simulink library "tm4c1294npdt"  (R2013b)
settings: Solver=ode45  StartTime=0.0  StopTime=10.0  RelTol=1e-3
libraries: tm4c1294npdt x2
settings Model: Creator=Q365198  LastModifiedBy=Q365198

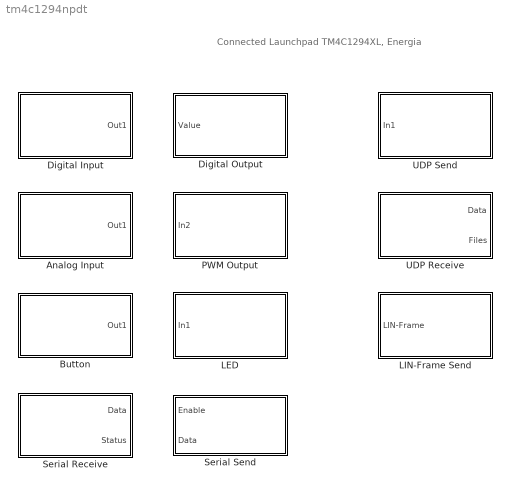
== system tm4c1294npdt ==
  note: Connected Launchpad TM4C1294XL, Energia
  Analog Input : Subsystem  mask(Energia Analog Input){popup_pin=14, pin=2, SampleTime=-1}
      mask prompts: popup_pin "Analog Input Pin:"; pin "Analog Pin"; SampleTime "Sample Time (-1 for inherited):"
      mask help:
      | Measure the voltage of a specified analog input pin. The block represents the voltage as a digital value (0-1023, minimum to maximum).
      |
      | Enter the number of the analog input pin. Do not assign the same pin number to multiple blocks within a model.
      mask TypeOptions popup_pin: 2 | 6 | 7 | 14 | 15 | 23 | 24 | 25 | 26 | 27 | 42 | 45 | 46 | 63 | 64 | 65 | 66 | 67 | 68 | 87
      mask Callback popup_pin:
      | thisBlock = gcb();
      | 
      | thisVarState = get_param(thisBlock, 'popup_pin');
      | set_param(thisBlock, 'pin', thisVarState);
      mask Display:
      | pic=imread('analogio.png');image(pic,[0.32 0.25 0.35 0.55]);
      | str = sprintf('Pin %i', pin);
      | text(0.5, 0.15, str, 'horizontalAlignment', 'center');
      | color('blue');
      | text(0.35, 0.87, 'TM4C1294XL', 'horizontalAlignment', 'left');
      | color('black');
  Button : Subsystem  mask(TM4C1294XL User Buttons){popup_pin=USR_SW1, pin=85, mode_popup=INPUT_PULLUP, mode=3, SampleTime=-1}
      mask prompts: popup_pin "User Button:"; pin "PinMode"; mode_popup "Input Mode:"; SampleTime "Sample Time (-1 for inherited):"
      mask help:
      | Read the logical value of a specified user Button on the TM4C1294XL Connected Launchpad.
      |
      | Choose available Buttons using the dropdown menu. Do not assign identical Buttons to more than one block (Fuctionality not guaranteed).
      mask TypeOptions popup_pin: USR_SW1 | USR_SW2
      mask Callback popup_pin:
      | thisBlock = gcb();
      | 
      | thisVarState = get_param(thisBlock, 'popup_pin');
      | if strcmp(thisVarState, 'USR_SW1')
      |     set_param(thisBlock, 'pin', '85');
      | elseif strcmp(thisVarState, 'USR_SW2')
      |     set_param(thisBlock, 'pin', '86');
      | end
      mask TypeOptions mode_popup: INPUT | INPUT_PULLDOWN | INPUT_PULLUP
      mask Callback mode_popup:
      | thisBlock = gcb();
      | 
      | thisVarState = get_param(thisBlock, 'mode_popup');
      | if strcmp(thisVarState, 'INPUT')
      |     set_param(thisBlock, 'mode', '1');
      | elseif strcmp(thisVarState, 'INPUT_PULLDOWN')
      |     set_param(thisBlock, 'mode', '2');
      | elseif strcmp(thisVarState, 'INPUT_PULLUP')
      |     set_param(thisBlock, 'mode', '3');
      | end
      mask Display:
      | pic=imread('push_button.jpg');image(pic,[0.32 0.20 0.35 0.55]);
      | str = sprintf('Pin %i', pin);
      | text(0.5, 0.15, str, 'horizontalAlignment', 'center');
      | color('blue');
      | text(0.35, 0.87, 'TM4C1294XL', 'horizontalAlignment', 'left');
      | color('black');
      | 
      | % Output Label
      | MaskValues=get_param(gcbh, 'MaskValues');
      | switch MaskValues{3}
      |     case 'INPUT'
      |         label = 'IN';
      |     case 'INPUT_PULLDOWN'
      |         label = 'IN_PD';
      |     case 'INPUT_PULLUP'
      |         label = 'IN_PU';
      |     otherwise
      |         label = '';
      | end
      | port_label('output',1,label);
  Digital Input : Subsystem  mask(Energia Digital Input){pin=2, mode_popup=INPUT, mode=1, SampleTime=-1}
      mask prompts: pin "Input Pin Number:"; mode_popup "Input Mode:"; SampleTime "Sample Time (-1 for inherited):"
      mask help:
      | Get the logical value of a specified digital input pin.
      |
      | Enter the number of the digital input pin. Do not assign the same pin number to multiple blocks within a model.
      mask TypeOptions mode_popup: INPUT | INPUT_PULLDOWN | INPUT_PULLUP
      mask Callback mode_popup:
      | thisBlock = gcb();
      | 
      | thisVarState = get_param(thisBlock, 'mode_popup');
      | if strcmp(thisVarState, 'INPUT')
      |     set_param(thisBlock, 'mode', '1');
      | elseif strcmp(thisVarState, 'INPUT_PULLDOWN')
      |     set_param(thisBlock, 'mode', '2');
      | elseif strcmp(thisVarState, 'INPUT_PULLUP')
      |     set_param(thisBlock, 'mode', '3');
      | end
      mask Display:
      | pic=imread('digitalio.png');image(pic,[0.32 0.25 0.35 0.55]);
      | str = sprintf('Pin %i', pin);
      | text(0.5, 0.15, str, 'horizontalAlignment', 'center');
      | color('blue');
      | text(0.35, 0.87, 'TM4C1294XL', 'horizontalAlignment', 'left');
      | color('black');
      | 
      | % Output Label
      | MaskValues=get_param(gcbh, 'MaskValues');
      | switch MaskValues{2}
      |     case 'INPUT'
      |         label = 'IN';
      |     case 'INPUT_PULLDOWN'
      |         label = 'IN_PD';
      |     case 'INPUT_PULLUP'
      |         label = 'IN_PU';
      | end
      | port_label('output',1,label);
  Digital Output : Subsystem  mask(Energia Digital Output){pin=82, SampleTime=-1}
      mask prompts: pin "Output Pin Number"; SampleTime "Sample Time (-1 for inherited):"
      mask help:
      | Set the logical value of a specified digital output pin.
      |
      | Enter the number of the digital output pin. Do not assign the same pin number to multiple blocks within a model.
      mask Display:
      | pic=imread('digitalio.png');image(pic,[0.32 0.25 0.35 0.55]);
      | str = sprintf('Pin %i', pin);
      | text(0.5, 0.15, str, 'horizontalAlignment', 'center');
      | color('blue');
      | text(0.35, 0.87, 'TM4C1294XL', 'horizontalAlignment', 'left');
      | color('black');
  LED : Subsystem  mask(TM4C1294XL User LEDs){popup_led=LED1, pin=81, SampleTime=-1}
      mask prompts: popup_led "User LEDs:"; SampleTime "Sample Time (-1 for inherited):"
      mask help:
      | Set the logical value of a specified user LED on the TM4C1294XL Connected Launchpad.
      |
      | Choose available LEDs using the dropdown menu. Do not assign identical LEDs to more than one block (Fuctionality not guaranteed).
      mask TypeOptions popup_led: LED1 | LED2 | LED3 | LED4
      mask Callback popup_led:
      | thisBlock = gcb();
      | 
      | thisVarState = get_param(thisBlock, 'popup_led');
      | if strcmp(thisVarState, 'LED1')
      |     set_param(thisBlock, 'pin', '81');
      | elseif strcmp(thisVarState, 'LED2')
      |     set_param(thisBlock, 'pin', '82');
      | elseif strcmp(thisVarState, 'LED3')
      |     set_param(thisBlock, 'pin', '83');
      | elseif strcmp(thisVarState, 'LED4')
      |     set_param(thisBlock, 'pin', '84');
      | end
      mask Display:
      | pic=imread('led_green.png');image(pic,[0.32 0.20 0.35 0.55]);
      | str = sprintf('Pin %i', pin);
      | text(0.5, 0.15, str, 'horizontalAlignment', 'center');
      | color('blue');
      | text(0.35, 0.87, 'TM4C1294XL', 'horizontalAlignment', 'left');
      | color('black');
  LIN-Frame Send : Subsystem  mask(LIN-Frame Send){portPopup=2, port=2, baudPopup=19200, baud=19200, txPin=57, SampleTime=-1}
      mask prompts: portPopup "Serial Port:"; baudPopup "Baudrate:"; SampleTime "Sample Time (-1 for inherited):"
      mask help:
      | This block is acutally sending complete LIN-Frames using baud speed and your defined UART port.
      |
      | REMEMBER: You have to input a byte stream which is representing a LIN-Frame but WITHOUT the "Break field".
      | -> The Bytestream should contain:
      | 1. Sync Field (0x55), 1 Byte
      | 2. Identifier (EventID, care about Parity), 1 Byte
      | 3. Databytes, 1 - 8 Bytes
      | 4. Checksum, 1 Byte
      mask TypeOptions portPopup: 2 | 3 | 4 | 5 | 6 | 7
      mask Callback portPopup:
      | thisBlock = gcb();
      | 
      | thisVarState = get_param(thisBlock, 'portPopup');
      | set_param(thisBlock, 'port', thisVarState);
      | 
      | switch thisVarState
      |     case '2'
      |         set_param(thisBlock, 'txPin', '57');
      |     case '3'
      |         set_param(thisBlock, 'txPin', '70');
      |     case '4'
      |         set_param(thisBlock, 'txPin', '66');
      |     case '5'
      |         set_param(thisBlock, 'txPin', '8');
      |     case '6'
      |         set_param(thisBlock, 'txPin', '44');
      |     case '7'
      |         set_param(thisBlock, 'txPin', '4');
      |     otherwise
      |         set_param(thisBlock, 'txPin', '57');
      | end
      mask TypeOptions baudPopup: 300 | 1200 | 2400 | 4800 | 9600 | 14400 | 19200 | 28800 | 38400 | 57600 | 76800 | 115200
      mask Callback baudPopup:
      | thisBlock = gcb();
      | 
      | thisVarState = get_param(thisBlock, 'baudPopup');
      | set_param(thisBlock, 'baud', thisVarState);
      mask Display:
      | pic=imread('Lin_Logo.jpg');image(pic,[0.50 0.10 0.45 0.65]);
      | 
      | color('blue');
      | text(0.38, 0.87, 'TM4C1294XL', 'horizontalAlignment', 'left');
      | 
      | color('red')
      | str = sprintf('UART%i',port);
      | text(0.02, 0.87, str,'horizontalAlignment', 'left');
      | color('black');
      | 
      | port_label('input', 1, 'LIN-Frame');
  PWM Output : Subsystem  mask(Energia PWM Output){popup_pin=7, pin=7, SampleTime=-1}
      mask prompts: popup_pin "PWM Output Pin:"; pin "PWM Output Pin:"; SampleTime "Sample Time (-1 for inherited):"
      mask help:
      | Generate square waveform on the specified analog output pin. The block input controls the duty cycle of the square waveform. An input value of 0 produces a 0 percent duty cycle, and an input value of 255 produces a 100 percent duty cycle. The frequency of the waveform is constant at approximately 490 Hz.
      |
      | Enter the number of the analog output pin (7, 9, 10, 14, 15, 19, 27-30, 35, 36, 42, 45, 46, 51, 57, 59, 69, 70, 75 - 77, 87, 90, 91). Do not assign the same pin number to multiple blocks within a model.
      mask TypeOptions popup_pin: 7 | 9 | 10 | 14 | 15 | 19 | 27 | 28 | 29 | 30 | 35 | 36 | 42 | 45 | 46 | 51 | 57 | 59 | 69 | 70 | 75 | 76 | 77 | 87 | 90 | 91
      mask Callback popup_pin:
      | thisBlock = gcb();
      | 
      | thisVarState = get_param(thisBlock, 'popup_pin');
      | set_param(thisBlock, 'pin', thisVarState);
      mask Display:
      | pic=imread('analogoutpwm.png');image(pic,[0.32 0.25 0.35 0.55]);
      | str = sprintf('Pin %i', pin);
      | text(0.5, 0.15, str, 'horizontalAlignment', 'center');
      | color('blue');
      | text(0.35, 0.87, 'TM4C1294XL', 'horizontalAlignment', 'left');
      | color('black');
  Serial Receive : Subsystem  mask(Energia Serial Receive){portPopup=1, port=1, baudPopup=9600, baud=9600, bufferSize=32, SampleTime=-1}
      mask prompts: portPopup "UART-Port (0 = flash/debug):"; baudPopup "Baudrate:"; bufferSize "Receive Buffer Size (1...64):"; SampleTime "Sample Time (-1 for inherited):"
      mask help:
      | Get bytes of data from the specified serial port and write it to the Data block output. Maximum Datasize can be defined (64 Bytes = Hardware Buffer).
      |
      | If data is received, Status block output gives the size of the received data. If data is not received, Status is equal 0.
      |
      | Do not assign the same port to more than one Serial Receive block. Please remeber that UART0 is normally used for debug/flash and external mode.
      mask TypeOptions portPopup: 0 | 1 | 2 | 3 | 4 | 5 | 6 | 7
      mask Callback portPopup:
      | thisBlock = gcb();
      | 
      | thisVarState = get_param(thisBlock, 'portPopup');
      | set_param(thisBlock, 'port', thisVarState);
      mask TypeOptions baudPopup: 300 | 1200 | 2400 | 4800 | 9600 | 14400 | 19200 | 28800 | 38400 | 57600 | 76800 | 115200
      mask Callback baudPopup:
      | thisBlock = gcb();
      | 
      | thisVarState = get_param(thisBlock, 'baudPopup');
      | set_param(thisBlock, 'baud', thisVarState);
      mask Display:
      | pic=imread('serial.png');image(pic,[0.28 0.18 0.45 0.65]);
      | 
      | str = sprintf('UART%i', (portPopup-1));
      | text(0.5, 0.15, str, 'horizontalAlignment', 'center');
      | color('blue');
      | text(0.35, 0.87, 'TM4C1294XL', 'horizontalAlignment', 'left');
      | color('black');
      | 
      | color('blue');
      | text(0.35, 0.87, 'TM4C1294XL', 'horizontalAlignment', 'left');
      | color('black');
      | 
      | str = sprintf('Data[%i]', bufferSize);
      | port_label('output', 1, str);
      | port_label('output', 2, 'Status');
  Serial Send : Subsystem  mask(Energia Serial Write){portPopup=1, port=1, baudPopup=9600, baud=9600, SampleTime=-1}
      mask prompts: portPopup "UART-Port (0 = flash/debug):"; baudPopup "Baudrate:"; SampleTime "SampleTime (-1 for inherited):"
      mask help:
      | Write bytes of data to the specified serial portt. Maximum Datasize should be 64 Bytes (Hardware Buffer).
      |
      | Do not assign the same port to more than one Serial Receive block. Please remeber that UART0 is normally used for debug/flash and external mode.
      mask TypeOptions portPopup: 0 | 1 | 2 | 3 | 4 | 5 | 6 | 7
      mask Callback portPopup:
      | thisBlock = gcb();
      | 
      | thisVarState = get_param(thisBlock, 'portPopup');
      | set_param(thisBlock, 'port', thisVarState);
      mask TypeOptions baudPopup: 300 | 1200 | 2400 | 4800 | 9600 | 14400 | 19200 | 28800 | 38400 | 57600 | 76800 | 115200
      mask Callback baudPopup:
      | thisBlock = gcb();
      | 
      | thisVarState = get_param(thisBlock, 'baudPopup');
      | set_param(thisBlock, 'baud', thisVarState);
      mask Display:
      | pic=imread('serial.png');image(pic,[0.28 0.18 0.45 0.65]);
      | 
      | str = sprintf('UART%i', (portPopup-1));
      | text(0.5, 0.15, str, 'horizontalAlignment', 'center');
      | color('blue');
      | text(0.35, 0.87, 'TM4C1294XL', 'horizontalAlignment', 'left');
      | color('black');
      | 
      | color('blue');
      | text(0.35, 0.87, 'TM4C1294XL', 'horizontalAlignment', 'left');
      | color('black');
      | 
      | str = sprintf('Data');
      | port_label('input', 2, str);
      | port_label('input', 1, 'Enable');
  UDP Receive : Subsystem  mask(Energia UDP Send){localPort=8000, simVectorSize=8, SampleTime=-1}
      mask prompts: localPort "Local Port:"; simVectorSize "Output Vector Size (1-500)"; SampleTime "Sample time (-1 for inherited):"
      mask help: Configure TCP/IP stack to send UDP messages to a remote interface identified by IP address and IP port pair.
      mask Display:
      | pic=imread('ethernetshield.png');image(pic,[0.32 0.25 0.35 0.55]);text(0.5, 0.15, 'Pin 9', 'horizontalAlignment', 'center');
      | color('blue');
      | text(0.35, 0.87, 'TM4C1294XL', 'horizontalAlignment', 'left');
      | color('black');
  UDP Send : Subsystem  mask(Energia UDP Send){remoteIPOctetString=192.168.0.5, remotePort=8888, localport=8000, remoteIP1=192, remoteIP2=168, remoteIP3=0, remoteIP4=5, SampleTime=-1}
      mask prompts: remoteIPOctetString "Remote IP Address:"; remotePort "Remote Port:"; localport "Local Port:"; remoteIP1 "Remote IP First"; remoteIP2 "Remote IP Second"; remoteIP3 "Remote IP Third"; remoteIP4 "Remote IP Fourth"; SampleTime "Sample time (-1 for inherited):"
      mask help: Configure TCP/IP stack to send UDP messages to a remote interface identified by IP address and IP port pair.
      mask Callback remoteIPOctetString:
      | thisBlock = gcb();
      | 
      | thisVarState = get_param(thisBlock, 'remoteIPOctetString');
      | parts = strsplit(thisVarState, '.');
      | set_param(thisBlock, 'remoteIP1', parts{1});
      | set_param(thisBlock, 'remoteIP2', parts{2});
      | set_param(thisBlock, 'remoteIP3', parts{3});
      | set_param(thisBlock, 'remoteIP4', parts{4});
      mask Display:
      | pic=imread('ethernetshield.png');image(pic,[0.32 0.25 0.35 0.55]);text(0.5, 0.15, 'Pin 9', 'horizontalAlignment', 'center');
      | color('blue');
      | text(0.35, 0.87, 'TM4C1294XL', 'horizontalAlignment', 'left');
      | color('black');

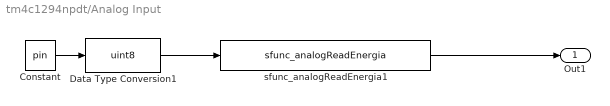
== system tm4c1294npdt/Analog Input ==
  Constant : Constant  Value=pin
  Data Type Conversion1 : DataTypeConversion  OutDataTypeStr=uint8  SaturateOnIntegerOverflow=on
  sfunc_analogReadEnergia1 : S-Function  FunctionName=sfunc_analogReadEnergia  Parameters=SampleTime  EnableBusSupport=off  mask(Legacy Function){SFunctionSpec=int16 y1 = analogReadEnergia(uint8 u1), SampleTime=SampleTime, ShowSpec=on}
      mask prompts: SampleTime "Sample time (-1 for inherited):"; ShowSpec "Display function specification"
      mask help:
      | This block allows you to call the legacy functions specified by the following Legacy Code Tool definition:
      | def.SFunctionName = 'sfunc_analogReadEnergia';
      | def.OutputFcnSpec = 'int16 y1 = analogReadEnergia(uint8 u1)';
      | def.HeaderFiles = {'gpioEnergia.h'};
      | def.SourceFiles = {'gpioEnergia.c'};
      | def.IncPaths = {'C:\MATLAB\SupportPackages\R2013b\TM4C1294NPDT\blocks\src\'};
      | def.SrcPaths = {'C:\MATLAB\SupportPackages\R2013b\TM4C1294NPDT\blocks\src\'};
      | def.SampleTime = 'parameterized';
      mask Help: <p>This block was generated automatically by the Legacy Code Tool. For detailed help on this tool, call<a href="matlab:legacy_code('help')"> legacy_code('help')</a>.</p>
      mask Callback ShowSpec:
      | if strcmp(get_param(gcbh, 'ShowSpec'), 'on')
      |   set_param(gcbh, 'MaskDisplay', sprintf('fprintf(''%s'');', get_param(gcbh, 'SFunctionSpec')));
      | else
      |   set_param(gcbh, 'MaskDisplay', sprintf('fprintf(''%s'');', get_param(gcbh, 'FunctionName')));
      | end
      mask Display: fprintf('int16 y1 = analogReadEnergia(uint8 u1)');
  Out1 : Outport
  wires:
  sfunc_analogReadEnergia1/1 -> Out1/1
  Constant/1 -> Data Type Conversion1/1
  Data Type Conversion1/1 -> sfunc_analogReadEnergia1/1

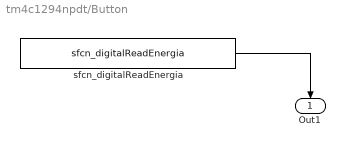
== system tm4c1294npdt/Button ==
  sfcn_digitalReadEnergia : tm4c1294npdt/Digital Input/sfcn_digitalReadEnergia  SFunctionSpec=uint8 y1 = digitalReadEnergia(uint8 p1)  SParameter1=pin  SParameter2=mode  SampleTime=SampleTime  ShowSpec=on
  Out1 : Outport
  wires:
  sfcn_digitalReadEnergia/1 -> Out1/1

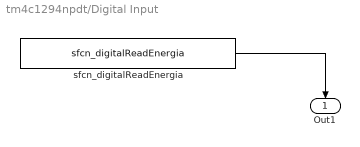
== system tm4c1294npdt/Digital Input ==
  sfcn_digitalReadEnergia : S-Function  FunctionName=sfcn_digitalReadEnergia  Parameters=SParameter1, SParameter2, SampleTime  EnableBusSupport=off  mask(Legacy Function){SFunctionSpec=uint8 y1 = digitalReadEnergia(uint8 p1), SParameter1=pin, SParameter2=mode, SampleTime=SampleTime, ShowSpec=on}
      mask prompts: SParameter1 "P1:"; SParameter2 "P2:"; SampleTime "Sample time (-1 for inherited):"; ShowSpec "Display function specification"
      mask help:
      | This block allows you to call the legacy functions specified by the following Legacy Code Tool definition:
      | def.SFunctionName = 'sfcn_digitalReadEnergia';
      | def.OutputFcnSpec = 'uint8 y1 = digitalReadEnergia(uint8 p1)';
      | def.StartFcnSpec = 'void digitalModeInitialize(uint8 p1, uint8 p2)';
      | def.HeaderFiles = {'gpioEnergia.h'};
      | def.SourceFiles = {'gpioEnergia.c'};
      | def.IncPaths = {'C:\MATLAB\SupportPackages\R2013b\TM4C1294NPDT\blocks\src\'};
      | def.SrcPaths = {'C:\MATLAB\SupportPackages\R2013b\TM4C1294NPDT\blocks\src\'};
      | def.SampleTime = 'parameterized';
      mask Help: <p>This block was generated automatically by the Legacy Code Tool. For detailed help on this tool, call<a href="matlab:legacy_code('help')"> legacy_code('help')</a>.</p>
      mask Callback ShowSpec:
      | if strcmp(get_param(gcbh, 'ShowSpec'), 'on')
      |   set_param(gcbh, 'MaskDisplay', sprintf('fprintf(''%s'');', get_param(gcbh, 'SFunctionSpec')));
      | else
      |   set_param(gcbh, 'MaskDisplay', sprintf('fprintf(''%s'');', get_param(gcbh, 'FunctionName')));
      | end
      mask Display: fprintf('uint8 y1 = digitalReadEnergia(uint8 p1)');
  Out1 : Outport
  wires:
  sfcn_digitalReadEnergia/1 -> Out1/1

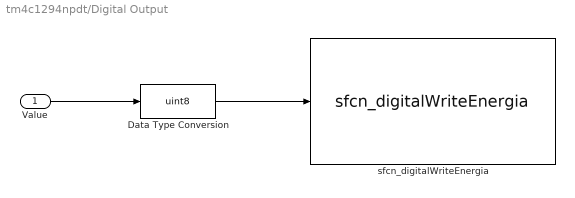
== system tm4c1294npdt/Digital Output ==
  Value : Inport
  Data Type Conversion : DataTypeConversion  OutDataTypeStr=uint8  SaturateOnIntegerOverflow=on
  sfcn_digitalWriteEnergia : S-Function  FunctionName=sfcn_digitalWriteEnergia  Parameters=SParameter1, SParameter2, SampleTime  EnableBusSupport=off  mask(Legacy Function){SFunctionSpec=void digitalWriteEnergia(uint8 p1, uint8 u1), SParameter1=pin, SParameter2=4, SampleTime=SampleTime, ShowSpec=on}
      mask prompts: SParameter1 "P1:"; SParameter2 "P2:"; SampleTime "Sample time (-1 for inherited):"; ShowSpec "Display function specification"
      mask help:
      | This block allows you to call the legacy functions specified by the following Legacy Code Tool definition:
      | def.SFunctionName = 'sfcn_digitalWriteEnergia';
      | def.OutputFcnSpec = 'void digitalWriteEnergia(uint8 p1, uint8 u1)';
      | def.StartFcnSpec = 'void digitalModeInitialize(uint8 p1, uint8 p2)';
      | def.HeaderFiles = {'gpioEnergia.h'};
      | def.SourceFiles = {'gpioEnergia.c'};
      | def.IncPaths = {'C:\MATLAB\SupportPackages\R2013b\TM4C1294NPDT\blocks\src\'};
      | def.SrcPaths = {'C:\MATLAB\SupportPackages\R2013b\TM4C1294NPDT\blocks\src\'};
      | def.SampleTime = 'parameterized';
      mask Help: <p>This block was generated automatically by the Legacy Code Tool. For detailed help on this tool, call<a href="matlab:legacy_code('help')"> legacy_code('help')</a>.</p>
      mask Callback ShowSpec:
      | if strcmp(get_param(gcbh, 'ShowSpec'), 'on')
      |   set_param(gcbh, 'MaskDisplay', sprintf('fprintf(''%s'');', get_param(gcbh, 'SFunctionSpec')));
      | else
      |   set_param(gcbh, 'MaskDisplay', sprintf('fprintf(''%s'');', get_param(gcbh, 'FunctionName')));
      | end
      mask Display: fprintf('void digitalWriteEnergia(uint8 p1, uint8 u1)');
  wires:
  Value/1 -> Data Type Conversion/1
  Data Type Conversion/1 -> sfcn_digitalWriteEnergia/1

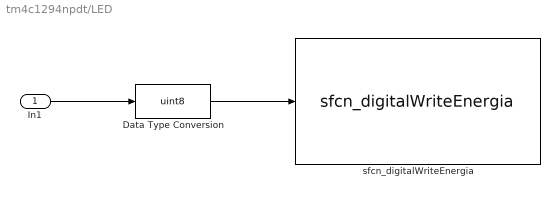
== system tm4c1294npdt/LED ==
  In1 : Inport
  Data Type Conversion : DataTypeConversion  OutDataTypeStr=uint8  SaturateOnIntegerOverflow=on
  sfcn_digitalWriteEnergia : tm4c1294npdt/Digital Output/sfcn_digitalWriteEnergia  SFunctionSpec=void digitalWriteEnergia(uint8 p1, uint8 u1)  SParameter1=pin  SParameter2=4  SampleTime=SampleTime  ShowSpec=on
  wires:
  In1/1 -> Data Type Conversion/1
  Data Type Conversion/1 -> sfcn_digitalWriteEnergia/1

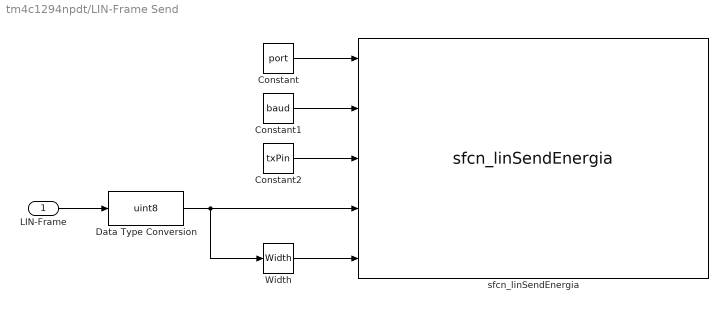
== system tm4c1294npdt/LIN-Frame Send ==
  LIN-Frame : Inport
  Constant : Constant  Value=port  OutDataTypeStr=int16
  Constant1 : Constant  Value=baud  OutDataTypeStr=int32
  Constant2 : Constant  Value=txPin  OutDataTypeStr=uint8
  Data Type Conversion : DataTypeConversion  OutDataTypeStr=uint8
  Width : Width  DataType=uint8
  sfcn_linSendEnergia : S-Function  FunctionName=sfcn_linSendEnergia  Parameters=SampleTime  EnableBusSupport=off  mask(Legacy Function){SFunctionSpec=void linSendEnergia(int16 u1, int32 u2, uint8 u3, uint8 u4[], uint8 u5), SampleTime=SampleTime, ShowSpec=on}
      mask prompts: SampleTime "Sample time (-1 for inherited):"; ShowSpec "Display function specification"
      mask help:
      | This block allows you to call the legacy functions specified by the following Legacy Code Tool definition:
      | def.SFunctionName = 'sfcn_linSendEnergia';
      | def.OutputFcnSpec = 'void linSendEnergia(int16 u1, int32 u2, uint8 u3, uint8 u4[], uint8 u5)';
      | def.HeaderFiles = {'serialEnergia.h'};
      | def.SourceFiles = {'serialEnergia.c'};
      | def.IncPaths = {'C:\MATLAB\SupportPackages\R2013b\TM4C1294NPDT\blocks\src\'};
      | def.SrcPaths = {'C:\MATLAB\SupportPackages\R2013b\TM4C1294NPDT\blocks\src\'};
      | def.SampleTime = 'parameterized';
      mask Help: <p>This block was generated automatically by the Legacy Code Tool. For detailed help on this tool, call<a href="matlab:legacy_code('help')"> legacy_code('help')</a>.</p>
      mask Callback ShowSpec:
      | if strcmp(get_param(gcbh, 'ShowSpec'), 'on')
      |   set_param(gcbh, 'MaskDisplay', sprintf('fprintf(''%s'');', get_param(gcbh, 'SFunctionSpec')));
      | else
      |   set_param(gcbh, 'MaskDisplay', sprintf('fprintf(''%s'');', get_param(gcbh, 'FunctionName')));
      | end
      mask Display: fprintf('void linSendEnergia(int16 u1, int32 u2, uint8 u3, uint8 u4[], uint8 u5)');
  wires:
  LIN-Frame/1 -> Data Type Conversion/1
  Constant/1 -> sfcn_linSendEnergia/1
  Constant1/1 -> sfcn_linSendEnergia/2
  Constant2/1 -> sfcn_linSendEnergia/3
  Width/1 -> sfcn_linSendEnergia/5
  Data Type Conversion/1 -> Width/1, sfcn_linSendEnergia/4

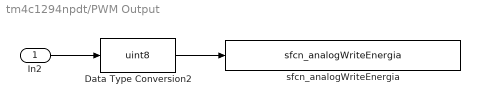
== system tm4c1294npdt/PWM Output ==
  In2 : Inport
  Data Type Conversion2 : DataTypeConversion  OutDataTypeStr=uint8  SampleTime=SampleTime  SaturateOnIntegerOverflow=on
  sfcn_analogWriteEnergia : S-Function  FunctionName=sfcn_analogWriteEnergia  Parameters=SParameter1, SParameter2, SampleTime  EnableBusSupport=off  mask(Legacy Function){SFunctionSpec=void analogWriteEnergia(uint8 p1, uint8 u1), SParameter1=pin, SParameter2=4, SampleTime=SampleTime, ShowSpec=on}
      mask prompts: SParameter1 "Pin:"; SParameter2 "Pin Mode (4=OUTPUT):"; SampleTime "Sample time (-1 for inherited):"; ShowSpec "Display function specification"
      mask help:
      | This block allows you to call the legacy functions specified by the following Legacy Code Tool definition:
      | def.SFunctionName = 'sfcn_analogWriteEnergia';
      | def.OutputFcnSpec = 'void analogWriteEnergia(uint8 p1, uint8 u1)';
      | def.StartFcnSpec = 'void digitalModeInitialize(uint8 p1, uint8 p2)';
      | def.HeaderFiles = {'gpioEnergia.h'};
      | def.SourceFiles = {'gpioEnergia.c'};
      | def.IncPaths = {'C:\MATLAB\SupportPackages\R2013b\TM4C1294NPDT\blocks\src\'};
      | def.SrcPaths = {'C:\MATLAB\SupportPackages\R2013b\TM4C1294NPDT\blocks\src\'};
      | def.SampleTime = 'parameterized';
      mask Help: <p>This block was generated automatically by the Legacy Code Tool. For detailed help on this tool, call<a href="matlab:legacy_code('help')"> legacy_code('help')</a>.</p>
      mask Callback ShowSpec:
      | if strcmp(get_param(gcbh, 'ShowSpec'), 'on')
      |   set_param(gcbh, 'MaskDisplay', sprintf('fprintf(''%s'');', get_param(gcbh, 'SFunctionSpec')));
      | else
      |   set_param(gcbh, 'MaskDisplay', sprintf('fprintf(''%s'');', get_param(gcbh, 'FunctionName')));
      | end
      mask Display: fprintf('void analogWriteEnergia(uint8 p1, uint8 u1)');
  wires:
  In2/1 -> Data Type Conversion2/1
  Data Type Conversion2/1 -> sfcn_analogWriteEnergia/1

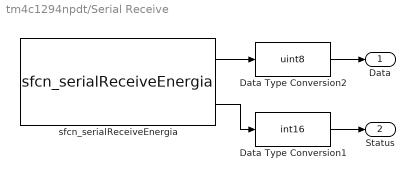
== system tm4c1294npdt/Serial Receive ==
  Data Type Conversion1 : DataTypeConversion  OutDataTypeStr=int16  SampleTime=SampleTime  SaturateOnIntegerOverflow=on
  Data Type Conversion2 : DataTypeConversion  OutDataTypeStr=uint8  SampleTime=SampleTime  SaturateOnIntegerOverflow=on
  sfcn_serialReceiveEnergia : S-Function  FunctionName=sfcn_serialReceiveEnergia  Parameters=SParameter1, SParameter2, SParameter3, SampleTime  EnableBusSupport=off  mask(Legacy Function){SFunctionSpec=void serialReceiveEnergia(int16 p1, uint8 y1[p3], int16 y2[1], int16 p3), SParameter1=port, SParameter2=baud, SParameter3=bufferSize, SampleTime=SampleTime, ShowSpec=on}
      mask prompts: SParameter1 "P1:"; SParameter2 "P2:"; SParameter3 "P3:"; SampleTime "Sample time (-1 for inherited):"; ShowSpec "Display function specification"
      mask help:
      | This block allows you to call the legacy functions specified by the following Legacy Code Tool definition:
      | def.SFunctionName = 'sfcn_serialReceiveEnergia';
      | def.OutputFcnSpec = 'void serialReceiveEnergia(int16 p1, uint8 y1[p3], int16 y2[1], int16 p3)';
      | def.StartFcnSpec = 'serialInitializeEnergia(int16 p1, int32 p2)';
      | def.HeaderFiles = {'serialEnergia.h'};
      | def.SourceFiles = {'serialEnergia.c'};
      | def.IncPaths = {'C:\MATLAB\SupportPackages\R2013b\TM4C1294NPDT\blocks\src\'};
      | def.SrcPaths = {'C:\MATLAB\SupportPackages\R2013b\TM4C1294NPDT\blocks\src\'};
      | def.SampleTime = 'parameterized';
      mask Help: <p>This block was generated automatically by the Legacy Code Tool. For detailed help on this tool, call<a href="matlab:legacy_code('help')"> legacy_code('help')</a>.</p>
      mask Callback ShowSpec:
      | if strcmp(get_param(gcbh, 'ShowSpec'), 'on')
      |   set_param(gcbh, 'MaskDisplay', sprintf('fprintf(''%s'');', get_param(gcbh, 'SFunctionSpec')));
      | else
      |   set_param(gcbh, 'MaskDisplay', sprintf('fprintf(''%s'');', get_param(gcbh, 'FunctionName')));
      | end
      mask Display: fprintf('void serialReceiveEnergia(int16 p1, uint8 y1[p3], int16 y2[1], int16 p3)');
  Data : Outport
  Status : Outport  Port=2
  wires:
  sfcn_serialReceiveEnergia/1 -> Data Type Conversion2/1
  sfcn_serialReceiveEnergia/2 -> Data Type Conversion1/1
  Data Type Conversion2/1 -> Data/1
  Data Type Conversion1/1 -> Status/1

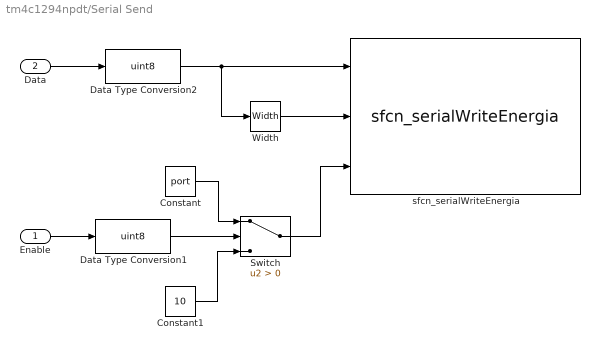
== system tm4c1294npdt/Serial Send ==
  Enable : Inport
  Data : Inport  Port=2
  Constant : Constant  Value=port  OutDataTypeStr=int16
  Constant1 : Constant  Value=10  OutDataTypeStr=int16
  Data Type Conversion1 : DataTypeConversion  OutDataTypeStr=uint8  SampleTime=SampleTime  SaturateOnIntegerOverflow=on
  Data Type Conversion2 : DataTypeConversion  OutDataTypeStr=uint8  SampleTime=SampleTime  SaturateOnIntegerOverflow=on
  Switch : Switch  Criteria=u2 > Threshold  OutDataTypeStr=int16
  Width : Width  DataType=int16
  sfcn_serialWriteEnergia : S-Function  FunctionName=sfcn_serialWriteEnergia  Parameters=SParameter1, SParameter2, SampleTime  EnableBusSupport=off  mask(Legacy Function){SFunctionSpec=void serialWriteEnergia(int16 u3, uint8 u1[], int16 u2), SParameter1=port, SParameter2=baud, SampleTime=SampleTime, ShowSpec=on}
      mask prompts: SParameter1 "P1:"; SParameter2 "P2:"; SampleTime "Sample time (-1 for inherited):"; ShowSpec "Display function specification"
      mask help:
      | This block allows you to call the legacy functions specified by the following Legacy Code Tool definition:
      | def.SFunctionName = 'sfcn_serialWriteEnergia';
      | def.OutputFcnSpec = 'void serialWriteEnergia(int16 u3, uint8 u1[], int16 u2)';
      | def.StartFcnSpec = 'serialInitializeEnergia(int16 p1, int32 p2)';
      | def.HeaderFiles = {'serialEnergia.h'};
      | def.SourceFiles = {'serialEnergia.c'};
      | def.IncPaths = {'C:\MATLAB\SupportPackages\R2013b\TM4C1294NPDT\blocks\src\'};
      | def.SrcPaths = {'C:\MATLAB\SupportPackages\R2013b\TM4C1294NPDT\blocks\src\'};
      | def.SampleTime = 'parameterized';
      mask Help: <p>This block was generated automatically by the Legacy Code Tool. For detailed help on this tool, call<a href="matlab:legacy_code('help')"> legacy_code('help')</a>.</p>
      mask Callback ShowSpec:
      | if strcmp(get_param(gcbh, 'ShowSpec'), 'on')
      |   set_param(gcbh, 'MaskDisplay', sprintf('fprintf(''%s'');', get_param(gcbh, 'SFunctionSpec')));
      | else
      |   set_param(gcbh, 'MaskDisplay', sprintf('fprintf(''%s'');', get_param(gcbh, 'FunctionName')));
      | end
      mask Display: fprintf('void serialWriteEnergia(int16 u3, uint8 u1[], int16 u2)');
  wires:
  Data/1 -> Data Type Conversion2/1
  Width/1 -> sfcn_serialWriteEnergia/2
  Data Type Conversion2/1 -> sfcn_serialWriteEnergia/1, Width/1
  Enable/1 -> Data Type Conversion1/1
  Data Type Conversion1/1 -> Switch/2
  Constant/1 -> Switch/1
  Switch/1 -> sfcn_serialWriteEnergia/3
  Constant1/1 -> Switch/3

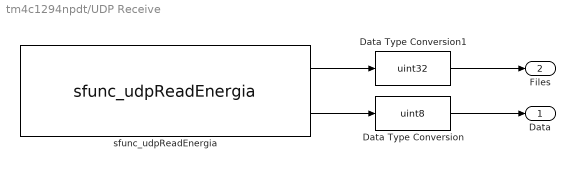
== system tm4c1294npdt/UDP Receive ==
  Data Type Conversion : DataTypeConversion  OutDataTypeStr=uint8  SaturateOnIntegerOverflow=on
  Data Type Conversion1 : DataTypeConversion  OutDataTypeStr=uint32  SaturateOnIntegerOverflow=on
  sfunc_udpReadEnergia : S-Function  FunctionName=sfunc_udpReadEnergia  Parameters=localPort, simVectorSize, SampleTime  EnableBusSupport=off  mask(Legacy Function){SFunctionSpec=int32 y1 = udpReadEnergia(uint8 y2[p2], uint32 p1, uint16 p2), ShowSpec=on}
      mask prompts: ShowSpec "Display function specification"
      mask help:
      | This block allows you to call the legacy functions specified by the following Legacy Code Tool definition:
      | def.SFunctionName = 'sfunc_udpReadEnergia';
      | def.OutputFcnSpec = 'int32 y1 = udpReadEnergia(uint8 y2[p2], uint32 p1, uint16 p2)';
      | def.HeaderFiles = {'ethernetEnergia.h'};
      | def.SourceFiles = {'ethernetEnergia.c'};
      | def.SampleTime = 'parameterized';
      mask Help: <p>This block was generated automatically by the Legacy Code Tool. For detailed help on this tool, call<a href="matlab:legacy_code('help')"> legacy_code('help')</a>.</p>
      mask Callback ShowSpec:
      | if strcmp(get_param(gcbh, 'ShowSpec'), 'on')
      |   set_param(gcbh, 'MaskDisplay', sprintf('fprintf(''%s'');', get_param(gcbh, 'SFunctionSpec')));
      | else
      |   set_param(gcbh, 'MaskDisplay', sprintf('fprintf(''%s'');', get_param(gcbh, 'FunctionName')));
      | end
      mask Display: fprintf('int32 y1 = udpReadEnergia(uint8 y2[p2], uint32 p1, uint16 p2)');
  Data : Outport
  Files : Outport  Port=2
  wires:
  Data Type Conversion1/1 -> Files/1
  sfunc_udpReadEnergia/1 -> Data Type Conversion1/1
  sfunc_udpReadEnergia/2 -> Data Type Conversion/1
  Data Type Conversion/1 -> Data/1

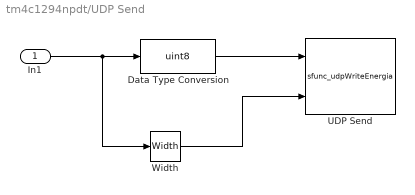
== system tm4c1294npdt/UDP Send ==
  In1 : Inport
  Data Type Conversion : DataTypeConversion  OutDataTypeStr=uint8  SaturateOnIntegerOverflow=on
  UDP Send : S-Function  FunctionName=sfunc_udpWriteEnergia  Parameters=localport, remotePort, remoteIP1, remoteIP2, remoteIP3, remoteIP4, SampleTime  EnableBusSupport=off  mask(Legacy Function){SFunctionSpec=udpWriteEnergia(uint8 u1[], uint32 p1, uint32 p2, uint8 p3, uint8 p4, uint8 p5 uint8 p6), ShowSpec=on}
      mask prompts: ShowSpec "Display function specification"
      mask help:
      | This block allows you to call the legacy functions specified by the following Legacy Code Tool definition:
      | def.SFunctionName = 'sfunc_udpWriteEnergia';
      | def.OutputFcnSpec = 'udpWriteEnergia(uint8 u1[], uint32 p1, uint32 p2, uint8 p3, uint8 p4, uint8 p5 uint8 p6)';
      | def.HeaderFiles = {'ethernetEnergia.h'};
      | def.SourceFiles = {'ethernetEnergia.c'};
      | def.SampleTime = 'parameterized';
      mask Help: <p>This block was generated automatically by the Legacy Code Tool. For detailed help on this tool, call<a href="matlab:legacy_code('help')"> legacy_code('help')</a>.</p>
      mask Callback ShowSpec:
      | if strcmp(get_param(gcbh, 'ShowSpec'), 'on')
      |   set_param(gcbh, 'MaskDisplay', sprintf('fprintf(''%s'');', get_param(gcbh, 'SFunctionSpec')));
      | else
      |   set_param(gcbh, 'MaskDisplay', sprintf('fprintf(''%s'');', get_param(gcbh, 'FunctionName')));
      | end
      mask Display: fprintf('udpWriteEnergia(uint8 u1[], uint32 p1, uint32 p2, uint8 p3, uint8 p4, uint8 p5 uint8 p6)');
  Width : Width  DataType=uint32
  wires:
  Width/1 -> UDP Send/2
  Data Type Conversion/1 -> UDP Send/1
  In1/1 -> Data Type Conversion/1, Width/1
